simulink model "lab3_03_gain"  (R2025b)
settings: Solver=ode45  StartTime=0.0  StopTime=10.0  MaxStep=0.01  RelTol=1e-6
settings Model: Creator=Boris  LastModifiedBy=Boris

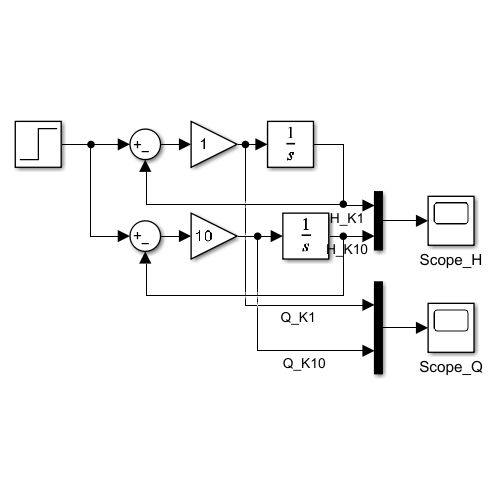
[thumbnail: Simulink's stored preview of the top-level diagram]
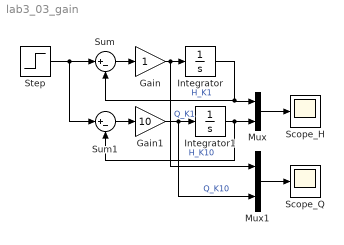
== system lab3_03_gain ==
  Gain : Gain
  Gain1 : Gain  Gain=10
  Integrator : Integrator
  Integrator1 : Integrator
  Mux : Mux  Inputs=2
  Mux1 : Mux  Inputs=2
  Scope_H : Scope
      settings: Tag=Scope_H  ActiveDisplayYMinimum=-14.766694195900916  ActiveDisplayYMaximum=18.142488903218592
  Scope_Q : Scope
      settings: Tag=Scope_H  ActiveDisplayYMinimum=-5.06764905178131  ActiveDisplayYMaximum=10.762230703101554
  Step : Step  SampleTime=0
  Sum : Sum  Inputs=|+-
  Sum1 : Sum  Inputs=|+-
  wires:
  Integrator/1 -> Mux/1, Sum/2  "H_K1"
  Step/1 -> Sum1/1, Sum/1
  Sum/1 -> Gain/1
  Gain/1 -> Mux1/1, Integrator/1  "Q_K1"
  Gain1/1 -> Mux1/2, Integrator1/1  "Q_K10"
  Sum1/1 -> Gain1/1
  Integrator1/1 -> Mux/2, Sum1/2  "H_K10"
  Mux/1 -> Scope_H/1
  Mux1/1 -> Scope_Q/1
